simulink model "pm4_motor"  (R2017a)
settings: Solver=VariableStepAuto  StartTime=0.0  StopTime=3.0  RelTol=1e-3
libraries: simulink x3
settings Model: Creator=robotica  LastModifiedBy=robotica

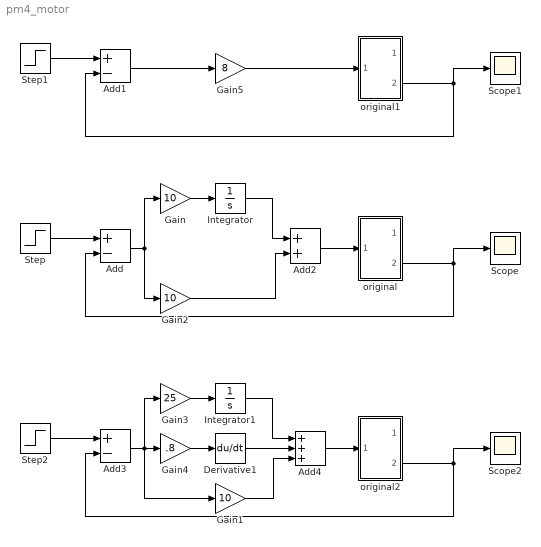
== system pm4_motor ==
  Add : Sum  Inputs=+-
  Add1 : Sum  Inputs=+-
  Add2 : Sum
  Add3 : Sum  Inputs=+-
  Add4 : Sum  Inputs=+++
  Derivative1 : Derivative
  Gain : Gain  Gain=10
  Gain1 : Gain  Gain=10
  Gain2 : Gain  Gain=10
  Gain3 : Gain  Gain=25
  Gain4 : Gain  Gain=.8
  Gain5 : Gain  Gain=8
  Integrator : Integrator
  Integrator1 : Integrator
  Scope : Scope
  Scope1 : Scope
  Scope2 : Scope
  Step : Step  SampleTime=1
  Step1 : Step  SampleTime=1
  Step2 : Step  SampleTime=1
  original : Subsystem
  original1 : Subsystem
  original2 : Subsystem
  wires:
  Step/1 -> Add/1
  original/2(clean) -> Add/2, Scope/1
  Gain/1 -> Integrator/1
  Integrator/1 -> Add2/1
  Add2/1 -> original/1(signal)
  Add/1 -> Gain2/1, Gain/1
  Gain2/1 -> Add2/2
  Step1/1 -> Add1/1
  original1/2(clean) -> Add1/2, Scope1/1
  Gain5/1 -> original1/1(signal)
  Add1/1 -> Gain5/1
  Add4/1 -> original2/1(signal)
  Gain4/1 -> Derivative1/1
  Step2/1 -> Add3/1
  Derivative1/1 -> Add4/2
  Gain3/1 -> Integrator1/1
  Integrator1/1 -> Add4/1
  original2/2(clean) -> Add3/2, Scope2/1
  Gain1/1 -> Add4/3
  Add3/1 -> Gain1/1, Gain4/1, Gain3/1

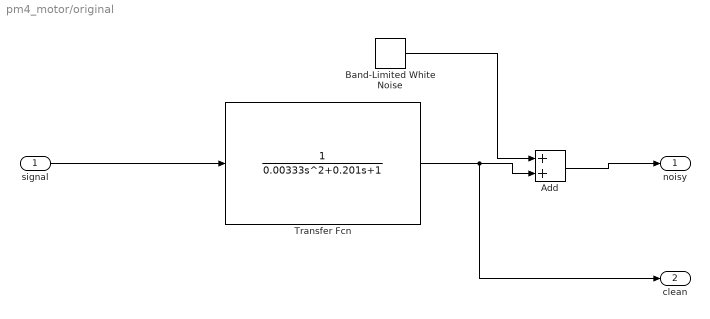
== system pm4_motor/original ==
  signal : Inport
  Add : Sum
  Band-Limited White Noise : simulink/Sources/Band-Limited White Noise  Cov=[0.0000001]  Ts=0.001  seed=[23341]
  Transfer Fcn : TransferFcn  Denominator=[0.00333 0.201 1]
  noisy : Outport
  clean : Outport  Port=2
  wires:
  Transfer Fcn/1 -> clean/1, Add/2
  Band-Limited White Noise/1 -> Add/1
  Add/1 -> noisy/1
  signal/1 -> Transfer Fcn/1

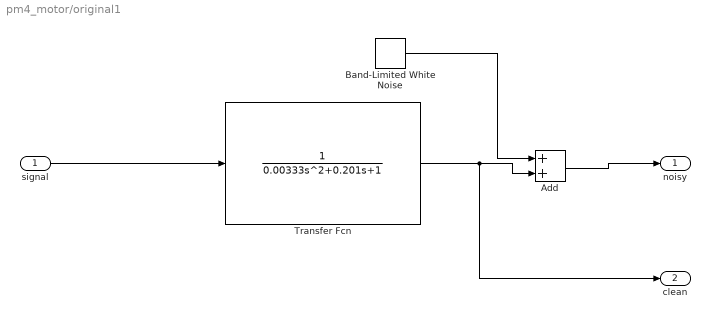
== system pm4_motor/original1 ==
  signal : Inport
  Add : Sum
  Band-Limited White Noise : simulink/Sources/Band-Limited White Noise  Cov=[0.0000001]  Ts=0.001  seed=[23341]
  Transfer Fcn : TransferFcn  Denominator=[0.00333 0.201 1]
  noisy : Outport
  clean : Outport  Port=2
  wires:
  Transfer Fcn/1 -> clean/1, Add/2
  Band-Limited White Noise/1 -> Add/1
  Add/1 -> noisy/1
  signal/1 -> Transfer Fcn/1

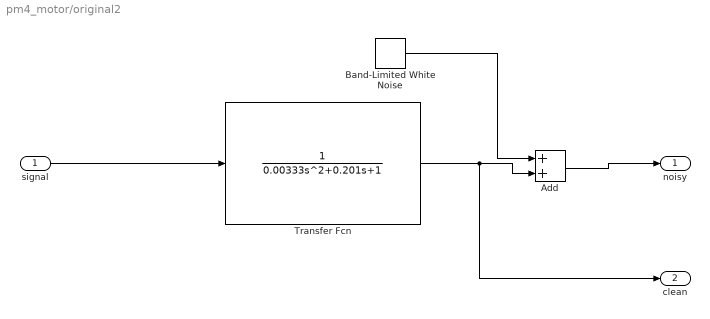
== system pm4_motor/original2 ==
  signal : Inport
  Add : Sum
  Band-Limited White Noise : simulink/Sources/Band-Limited White Noise  Cov=[0.0000001]  Ts=0.001  seed=[23341]
  Transfer Fcn : TransferFcn  Denominator=[0.00333 0.201 1]
  noisy : Outport
  clean : Outport  Port=2
  wires:
  Transfer Fcn/1 -> clean/1, Add/2
  Band-Limited White Noise/1 -> Add/1
  Add/1 -> noisy/1
  signal/1 -> Transfer Fcn/1
